simulink model "Marine_LocoMotive_UAV_est_git"  (R2018a)
settings: Solver=ode4  StartTime=0.0  StopTime=40  FixedStep=T  MaxStep=2*T  MinStep=T  RelTol=1e-4
values from neighbouring files (symbols this model uses):
  a_11 = 0.05*m_b    (= 0.625)    [Marine_LocoMotive_UAV_est_git_parameters.m]    (also in Marine_LocoMotive_UAV_medium_est_git_parameters.m = 1.6875; heave_dynamics_chart.m)
  a_33 = m_b    (= 12.5)    [Marine_LocoMotive_UAV_est_git_parameters.m]    (also in Marine_LocoMotive_UAV_medium_est_git_parameters.m = 33.75; heave_dynamics_chart.m)
  A_w = 1*3.3/2    (= 1.65)    [Marine_LocoMotive_UAV_est_git_parameters.m]    (also in Marine_LocoMotive_UAV_medium_est_git_parameters.m = 0.6)
  A_w2 = 1*1.2/2    (= 0.6)    [Marine_LocoMotive_UAV_est_git_parameters.m]    (also in Marine_LocoMotive_UAV_medium_est_git_parameters.m = 0.305)
  Ac = 0.0331    [Marine_LocoMotive_UAV_est_git_parameters.m]    (also in Marine_LocoMotive_UAV_medium_est_git_parameters.m = 0.422)
  alpha_bar = pi/4    (= 0.785398163397)    [Marine_LocoMotive_UAV_est_git_parameters.m]    (also in Marine_LocoMotive_UAV_medium_est_git_parameters.m; heave_dynamics_chart.m = pi/4*sign(V_bar(j)))
  Am = sysd.denominator{1}    [Marine_LocoMotive_UAV_est_git_parameters.m]    (also in Marine_LocoMotive_UAV_medium_est_git_parameters.m)
  Am1_LPF = sysd.denominator{1}    [Marine_LocoMotive_UAV_est_git_parameters.m]    (also in Marine_LocoMotive_UAV_medium_est_git_parameters.m)
  Am2_LPF = sysd.denominator{1}    [Marine_LocoMotive_UAV_est_git_parameters.m]    (also in Marine_LocoMotive_UAV_medium_est_git_parameters.m)
  Am_asw_LPF = sysd.denominator{1}    [Marine_LocoMotive_UAV_est_git_parameters.m]    (also in Marine_LocoMotive_UAV_medium_est_git_parameters.m)
  Am_coup_LPF = sysd.denominator{1}    [Marine_LocoMotive_UAV_est_git_parameters.m]    (also in Marine_LocoMotive_UAV_medium_est_git_parameters.m)
  Am_fast_coup_LPF = sysd.denominator{1}    [Marine_LocoMotive_UAV_est_git_parameters.m]    (also in Marine_LocoMotive_UAV_medium_est_git_parameters.m)
  Am_rdeL_LPF = sysd.denominator{1}    [Marine_LocoMotive_UAV_est_git_parameters.m]    (also in Marine_LocoMotive_UAV_medium_est_git_parameters.m)
  Am_reL_LPF = sysd.denominator{1}    [Marine_LocoMotive_UAV_est_git_parameters.m]    (also in Marine_LocoMotive_UAV_medium_est_git_parameters.m)
  Am_rref20_LPF = sysd.denominator{1}    [Marine_LocoMotive_UAV_est_git_parameters.m]    (also in Marine_LocoMotive_UAV_medium_est_git_parameters.m)
  Am_rref_LPF = sysd.denominator{1}    [Marine_LocoMotive_UAV_est_git_parameters.m]    (also in Marine_LocoMotive_UAV_medium_est_git_parameters.m)
  AmAlpha_LPF = sysd.denominator{1}    [Marine_LocoMotive_UAV_est_git_parameters.m]    (also in Marine_LocoMotive_UAV_medium_est_git_parameters.m)
  Amp_sf = 3    [Marine_LocoMotive_UAV_est_git_parameters.m]    (also in Marine_LocoMotive_UAV_medium_est_git_parameters.m)
  Amp_sf_rp = 0.05*m_u*g    (= 0.8829)    [Marine_LocoMotive_UAV_est_git_parameters.m]    (also in Marine_LocoMotive_UAV_medium_est_git_parameters.m = 9.56475)
  AmV_LPF = sysd.denominator{1}    [Marine_LocoMotive_UAV_est_git_parameters.m]    (also in Marine_LocoMotive_UAV_medium_est_git_parameters.m)
  AmZ_LPF = sysd.denominator{1}    [Marine_LocoMotive_UAV_est_git_parameters.m]    (also in Marine_LocoMotive_UAV_medium_est_git_parameters.m)
  b_11 = 0    [Marine_LocoMotive_UAV_est_git_parameters.m]    (also in Marine_LocoMotive_UAV_medium_est_git_parameters.m; heave_dynamics_chart.m)
  b_33 = 2*m_b*omega_h    (= 19.6349540849)    [Marine_LocoMotive_UAV_est_git_parameters.m]    (also in Marine_LocoMotive_UAV_medium_est_git_parameters.m = 84.8230016469; buoyancy_calc.m = 4.18879020479; heave_dynamics_chart.m = 2*m_b*omega_h)
  Bm = sysd.numerator{1}    [Marine_LocoMotive_UAV_est_git_parameters.m]    (also in Marine_LocoMotive_UAV_medium_est_git_parameters.m)
  Bm1_LPF = sysd.numerator{1}    [Marine_LocoMotive_UAV_est_git_parameters.m]    (also in Marine_LocoMotive_UAV_medium_est_git_parameters.m)
  Bm2_LPF = sysd.numerator{1}    [Marine_LocoMotive_UAV_est_git_parameters.m]    (also in Marine_LocoMotive_UAV_medium_est_git_parameters.m)
  Bm_asw_LPF = sysd.numerator{1}    [Marine_LocoMotive_UAV_est_git_parameters.m]    (also in Marine_LocoMotive_UAV_medium_est_git_parameters.m)
  Bm_coup_LPF = sysd.numerator{1}    [Marine_LocoMotive_UAV_est_git_parameters.m]    (also in Marine_LocoMotive_UAV_medium_est_git_parameters.m)
  Bm_fast_coup_LPF = sysd.numerator{1}    [Marine_LocoMotive_UAV_est_git_parameters.m]    (also in Marine_LocoMotive_UAV_medium_est_git_parameters.m)
  Bm_rdeL_LPF = sysd.numerator{1}    [Marine_LocoMotive_UAV_est_git_parameters.m]    (also in Marine_LocoMotive_UAV_medium_est_git_parameters.m)
  Bm_reL_LPF = sysd.numerator{1}    [Marine_LocoMotive_UAV_est_git_parameters.m]    (also in Marine_LocoMotive_UAV_medium_est_git_parameters.m)
  Bm_rref20_LPF = sysd.numerator{1}    [Marine_LocoMotive_UAV_est_git_parameters.m]    (also in Marine_LocoMotive_UAV_medium_est_git_parameters.m)
  Bm_rref_LPF = sysd.numerator{1}    [Marine_LocoMotive_UAV_est_git_parameters.m]    (also in Marine_LocoMotive_UAV_medium_est_git_parameters.m)
  BmAlpha_LPF = sysd.numerator{1}    [Marine_LocoMotive_UAV_est_git_parameters.m]    (also in Marine_LocoMotive_UAV_medium_est_git_parameters.m)
  BmV_LPF = sysd.numerator{1}    [Marine_LocoMotive_UAV_est_git_parameters.m]    (also in Marine_LocoMotive_UAV_medium_est_git_parameters.m)
  BmZ_LPF = sysd.numerator{1}    [Marine_LocoMotive_UAV_est_git_parameters.m]    (also in Marine_LocoMotive_UAV_medium_est_git_parameters.m)
  C_S = [5;9]*10^-3    [Marine_LocoMotive_UAV_est_git_parameters.m]    (also in Marine_LocoMotive_UAV_medium_est_git_parameters.m; heave_dynamics_chart.m = 0.075/(log10(Re)-2)^2)
  Cd_u = 0.2    [Marine_LocoMotive_UAV_est_git_parameters.m]    (also in Marine_LocoMotive_UAV_medium_est_git_parameters.m)
  D_x = b_11 + D_s(1)    [Marine_LocoMotive_UAV_est_git_parameters.m]    (also in Marine_LocoMotive_UAV_medium_est_git_parameters.m; heave_dynamics_chart.m = b_11 + D_s(i,j))
  D_z = b_33 + D_s(2)    [Marine_LocoMotive_UAV_est_git_parameters.m]    (also in Marine_LocoMotive_UAV_medium_est_git_parameters.m; heave_dynamics_chart.m)
  dc_M_p = 6.7    [Marine_LocoMotive_UAV_est_git_parameters.m]    (also in Marine_LocoMotive_UAV_medium_est_git_parameters.m)
  Delta_h = (A_im/A_b-0.5)*h_b    (= -0.0625)    [Marine_LocoMotive_UAV_est_git_parameters.m]    (also in Marine_LocoMotive_UAV_medium_est_git_parameters.m = -0.075; heave_dynamics_chart.m)
  eps_V = 0.1    [Marine_LocoMotive_UAV_est_git_parameters.m]    (also in Marine_LocoMotive_UAV_medium_est_git_parameters.m)
  epsilon_1 = 5    [Marine_LocoMotive_UAV_est_git_parameters.m]    (also in Marine_LocoMotive_UAV_medium_est_git_parameters.m)
  epsilon_e_u1 = 0.05    [Marine_LocoMotive_UAV_est_git_parameters.m]    (also in Marine_LocoMotive_UAV_medium_est_git_parameters.m)
  epsilon_w = 0    [Marine_LocoMotive_UAV_est_git_parameters.m]    (also in Marine_LocoMotive_UAV_medium_est_git_parameters.m)
  epsilon_w2 = pi    (= 3.14159265359)    [Marine_LocoMotive_UAV_est_git_parameters.m]    (also in Marine_LocoMotive_UAV_medium_est_git_parameters.m)
  g = 9.81    [Marine_LocoMotive_UAV_est_git_parameters.m]    (also in Marine_LocoMotive_UAV_medium_est_git_parameters.m; heave_dynamics_chart.m)
  gamma_d_p = (2*0.3/0.03*2*0.2*12/4)/10    (= 2.4)    [Marine_LocoMotive_UAV_est_git_parameters.m]    (also in Marine_LocoMotive_UAV_medium_est_git_parameters.m)
  H = 10    [Marine_LocoMotive_UAV_est_git_parameters.m]    (also in Marine_LocoMotive_UAV_medium_est_git_parameters.m)
  h_b = 0.25    [Marine_LocoMotive_UAV_est_git_parameters.m]    (also in Marine_LocoMotive_UAV_medium_est_git_parameters.m = 0.3; buoyancy_calc.m = 0.15; heave_dynamics_chart.m)
  J_b = m_b*h_b*l_b/12    (= 0.208333333333)    [Marine_LocoMotive_UAV_est_git_parameters.m]    (also in Marine_LocoMotive_UAV_medium_est_git_parameters.m = 1.265625; heave_dynamics_chart.m)
  J_u = 0.03    [Marine_LocoMotive_UAV_est_git_parameters.m]    (also in Marine_LocoMotive_UAV_medium_est_git_parameters.m = 1.51708333333)
  K = 40    [Marine_LocoMotive_UAV_est_git_parameters.m]    (also in Marine_LocoMotive_UAV_medium_est_git_parameters.m = 83.3333333333)
  k3 = 24    [Marine_LocoMotive_UAV_est_git_parameters.m]    (also in Marine_LocoMotive_UAV_medium_est_git_parameters.m)
  k4 = 0.8    [Marine_LocoMotive_UAV_est_git_parameters.m]    (also in Marine_LocoMotive_UAV_medium_est_git_parameters.m)
  k_w = omega_w^2/g    (= 0.0628797426165)    [Marine_LocoMotive_UAV_est_git_parameters.m]    (also in Marine_LocoMotive_UAV_medium_est_git_parameters.m = 0.160972141098; heave_dynamics_chart.m = omega_w^2/g)
  k_w2 = omega_w2^2/g    (= 0.160972141098)    [Marine_LocoMotive_UAV_est_git_parameters.m]    (also in Marine_LocoMotive_UAV_medium_est_git_parameters.m = 0.251518970466)
  kd_a = 5.6    [Marine_LocoMotive_UAV_est_git_parameters.m]    (also in Marine_LocoMotive_UAV_medium_est_git_parameters.m)
  kd_r = 19.5    [Marine_LocoMotive_UAV_est_git_parameters.m]    (also in Marine_LocoMotive_UAV_medium_est_git_parameters.m)
  kd_t = 10    [Marine_LocoMotive_UAV_est_git_parameters.m]    (also in Marine_LocoMotive_UAV_medium_est_git_parameters.m = 25)
  kd_x = 5    [Marine_LocoMotive_UAV_est_git_parameters.m]    (also in Marine_LocoMotive_UAV_medium_est_git_parameters.m)
  kd_z = 2    [Marine_LocoMotive_UAV_est_git_parameters.m]    (also in Marine_LocoMotive_UAV_medium_est_git_parameters.m)
  ki_a = 1.6    [Marine_LocoMotive_UAV_est_git_parameters.m]    (also in Marine_LocoMotive_UAV_medium_est_git_parameters.m)
  ki_r = 9    [Marine_LocoMotive_UAV_est_git_parameters.m]    (also in Marine_LocoMotive_UAV_medium_est_git_parameters.m)
  ki_T = 12    [Marine_LocoMotive_UAV_est_git_parameters.m]    (also in Marine_LocoMotive_UAV_medium_est_git_parameters.m)
  ki_x = 1.2    [Marine_LocoMotive_UAV_est_git_parameters.m]    (also in Marine_LocoMotive_UAV_medium_est_git_parameters.m)
  ki_z = 1    [Marine_LocoMotive_UAV_est_git_parameters.m]    (also in Marine_LocoMotive_UAV_medium_est_git_parameters.m)
  kp_a = 9.6    [Marine_LocoMotive_UAV_est_git_parameters.m]    (also in Marine_LocoMotive_UAV_medium_est_git_parameters.m)
  kp_r = 45    [Marine_LocoMotive_UAV_est_git_parameters.m]    (also in Marine_LocoMotive_UAV_medium_est_git_parameters.m)
  kp_t = 20    [Marine_LocoMotive_UAV_est_git_parameters.m]    (also in Marine_LocoMotive_UAV_medium_est_git_parameters.m = 50)
  kp_T = 25    [Marine_LocoMotive_UAV_est_git_parameters.m]    (also in Marine_LocoMotive_UAV_medium_est_git_parameters.m)
  kp_x = 7    [Marine_LocoMotive_UAV_est_git_parameters.m]    (also in Marine_LocoMotive_UAV_medium_est_git_parameters.m)
  kp_z = 3    [Marine_LocoMotive_UAV_est_git_parameters.m]    (also in Marine_LocoMotive_UAV_medium_est_git_parameters.m)
  L = 0.2    [Marine_LocoMotive_UAV_est_git_parameters.m]    (also in Marine_LocoMotive_UAV_medium_est_git_parameters.m = 0.8)
  l_b = 0.8    [Marine_LocoMotive_UAV_est_git_parameters.m]    (also in Marine_LocoMotive_UAV_medium_est_git_parameters.m = 1.5; buoyancy_calc.m = 0.5; heave_dynamics_chart.m)
  Lc_0 = 7    [Marine_LocoMotive_UAV_est_git_parameters.m]    (also in Marine_LocoMotive_UAV_medium_est_git_parameters.m = 20)
  LIMIT_CMD_PITCH = 45*pi/180    (= 0.785398163397)    [Marine_LocoMotive_UAV_est_git_parameters.m]    (also in Marine_LocoMotive_UAV_medium_est_git_parameters.m)
  LIMIT_uCMD_HEIGHT = 0.9*n_motors*K    (= 144)    [Marine_LocoMotive_UAV_est_git_parameters.m]    (also in Marine_LocoMotive_UAV_medium_est_git_parameters.m = 450)
  m_b = rho_w*Vol_b/4    (= 12.5)    [Marine_LocoMotive_UAV_est_git_parameters.m]    (also in Marine_LocoMotive_UAV_medium_est_git_parameters.m = 33.75; buoyancy_calc.m = 5; heave_dynamics_chart.m)
  m_u = 1.8    [Marine_LocoMotive_UAV_est_git_parameters.m]    (also in Marine_LocoMotive_UAV_medium_est_git_parameters.m = 19.5)
  min_sf = 5    [Marine_LocoMotive_UAV_est_git_parameters.m]    (also in Marine_LocoMotive_UAV_medium_est_git_parameters.m)
  min_sf_rp = 0.35*m_u*g    (= 6.1803)    [Marine_LocoMotive_UAV_est_git_parameters.m]    (also in Marine_LocoMotive_UAV_medium_est_git_parameters.m = 66.95325)
  n_motors = 4    [Marine_LocoMotive_UAV_est_git_parameters.m]    (also in Marine_LocoMotive_UAV_medium_est_git_parameters.m = 6)
  nu_w = 1.787*10^-6    (= 1.787e-06)    [Marine_LocoMotive_UAV_est_git_parameters.m]    (also in Marine_LocoMotive_UAV_medium_est_git_parameters.m; buoyancy_calc.m; heave_dynamics_chart.m)
  omega_w = 2*pi/T_w    (= 0.785398163397)    [Marine_LocoMotive_UAV_est_git_parameters.m]    (also in Marine_LocoMotive_UAV_medium_est_git_parameters.m = 1.25663706144; heave_dynamics_chart.m = 2*pi/T_i)
  omega_w2 = 2*pi/T_w2    (= 1.25663706144)    [Marine_LocoMotive_UAV_est_git_parameters.m]    (also in Marine_LocoMotive_UAV_medium_est_git_parameters.m = 1.57079632679)
  r_0 = sqrt( (X0_b(1) - X0_u(1))^2 +(X0_b(2) - X0_u(2))^2 )    [Marine_LocoMotive_UAV_est_git_parameters.m]    (also in Marine_LocoMotive_UAV_medium_est_git_parameters.m)
  R_b = 0.1    [buoyancy_calc.m]
  r_bar = Lc_0-0.3    (= 6.7)    [Marine_LocoMotive_UAV_est_git_parameters.m]    (also in Marine_LocoMotive_UAV_medium_est_git_parameters.m = 19.7)
  r_min = (zu_bar-H)-0.2    [Marine_LocoMotive_UAV_est_git_parameters.m]    (also in Marine_LocoMotive_UAV_medium_est_git_parameters.m)
  rho_a = 1.225    [Marine_LocoMotive_UAV_est_git_parameters.m]    (also in Marine_LocoMotive_UAV_medium_est_git_parameters.m)
  rho_w = 1000    [Marine_LocoMotive_UAV_est_git_parameters.m]    (also in Marine_LocoMotive_UAV_medium_est_git_parameters.m; buoyancy_calc.m; heave_dynamics_chart.m)
  T = 1/500    (= 0.002)    [Marine_LocoMotive_UAV_est_git_parameters.m]    (also in Marine_LocoMotive_UAV_medium_est_git_parameters.m)
  T_init = 10    [Marine_LocoMotive_UAV_est_git_parameters.m]    (also in Marine_LocoMotive_UAV_medium_est_git_parameters.m)
  Theta0 = 0    [Marine_LocoMotive_UAV_est_git_parameters.m]    (also in Marine_LocoMotive_UAV_medium_est_git_parameters.m)
  torque_corr = 2*cosd(60)+1    [Marine_LocoMotive_UAV_est_git_parameters.m]    (also in Marine_LocoMotive_UAV_medium_est_git_parameters.m)
  u_s = w_dir*A_w^2*omega_w*k_w*exp(2*k_w*(-Delta_h/2))    [Marine_LocoMotive_UAV_est_git_parameters.m]    (also in Marine_LocoMotive_UAV_medium_est_git_parameters.m)
  u_s2 = w_dir2*A_w2^2*omega_w2*k_w2*exp(2*k_w2*(-Delta_h/2))    [Marine_LocoMotive_UAV_est_git_parameters.m]    (also in Marine_LocoMotive_UAV_medium_est_git_parameters.m)
  u_t = -1*0.5*1    (= -0.5)    [Marine_LocoMotive_UAV_est_git_parameters.m]    (also in Marine_LocoMotive_UAV_medium_est_git_parameters.m)
  u_w = 0*0.2    (= 0)    [Marine_LocoMotive_UAV_est_git_parameters.m]    (also in Marine_LocoMotive_UAV_medium_est_git_parameters.m)
  V0_b = [u_t+u_w+u_s+v_x_w, v_z_w].*[1 1]    [Marine_LocoMotive_UAV_est_git_parameters.m]    (also in Marine_LocoMotive_UAV_medium_est_git_parameters.m = [u_t+u_w+u_s+v_x_w, v_z_w])
  V0_u = V0_b    [Marine_LocoMotive_UAV_est_git_parameters.m]    (also in Marine_LocoMotive_UAV_medium_est_git_parameters.m = [0 0])
  V_bar = 4    [Marine_LocoMotive_UAV_est_git_parameters.m]    (also in Marine_LocoMotive_UAV_medium_est_git_parameters.m; heave_dynamics_chart.m = [-20:0.1:20]')
  Vol_b = A_b*l_b    (= 0.05)    [Marine_LocoMotive_UAV_est_git_parameters.m]    (also in Marine_LocoMotive_UAV_medium_est_git_parameters.m = 0.135; heave_dynamics_chart.m)
  w_dir = 1    [Marine_LocoMotive_UAV_est_git_parameters.m]    (also in Marine_LocoMotive_UAV_medium_est_git_parameters.m; heave_dynamics_chart.m)
  w_dir2 = 1    [Marine_LocoMotive_UAV_est_git_parameters.m]    (also in Marine_LocoMotive_UAV_medium_est_git_parameters.m)
  X0_b = [0,H-Delta_h]    [Marine_LocoMotive_UAV_est_git_parameters.m]    (also in Marine_LocoMotive_UAV_medium_est_git_parameters.m)
  X0_u = X0_b + [3/7 3/7]*Lc_0    [Marine_LocoMotive_UAV_est_git_parameters.m]    (also in Marine_LocoMotive_UAV_medium_est_git_parameters.m)
  zu_bar = X0_b(2) + Lc_0*sin(alpha_bar_0)    [Marine_LocoMotive_UAV_est_git_parameters.m]    (also in Marine_LocoMotive_UAV_medium_est_git_parameters.m)
undefined symbols (not defined in the file or in its folder): Am_HPF, Am_LPF, Am_LPF2, an1, an1_v, an2, an3, Bm_HPF, Bm_LPF, Bm_LPF2, bn1, bn1_v, bn2, bn3, DiscIntNeverNeededParam, F, Light, magnitude, MIL, OMEGA_FILTER_OUTER, Tc, Tg, Tn, Ts, Tsc, Tz, X_GPS_offset
libraries: simulink x55, simulink_extras x9, aerolibwind2 x2
(part 8 of 9)

== system Marine_LocoMotive_UAV_est_git/UAV controller/u_a_Lyapunov/Subsystem1/alpha 0 ==
  X : Inport
  Trigger : TriggerPort  VariantControl=Variant
  Xu_init : Outport
  wires:
  X/1 -> Xu_init/1

== system Marine_LocoMotive_UAV_est_git/UAV controller/u_a_Lyapunov/Subsystem1/cond1 ==
  r : Inport
  r_dot : Inport  Port=2
  coupled : Inport  Port=3
  Constant : Constant  Value=Lc_0
  Constant2 : Constant  Value=T
  MATLAB Function : MATLAB Function  TreatAsAtomicUnit=on
  r_dot filt2 : Scope
  key : Outport
  wires:
  r/1 -> MATLAB Function/1(r)
  Constant/1 -> MATLAB Function/4(Lc)
  Constant2/1 -> MATLAB Function/5(dt)
  MATLAB Function/1(y) -> key/1
  r_dot/1 -> MATLAB Function/2(r_dot)
  coupled/1 -> MATLAB Function/3(coupled)
  MATLAB Function/2(t) -> r_dot filt2/1

== system Marine_LocoMotive_UAV_est_git/UAV controller/u_r_V_Lyapunov buoy velocity/Smooth channel switching1/C1 transition ==
  C1 : Inport
  switch : Inport  Port=2
  C2_0 : Inport  Port=3
  Compare To Constant : simulink/Logic and Bit Operations/Compare To Constant  relop=<  const=0.01  OutDataTypeStr=boolean
  Constant : Constant
  Constant1 : Constant  Value=0.01
  Delay1 : Delay  DelayLength=1
  IC : InitialCondition  Value=0
  Logical Operator : Logic  Operator=NOT  AllPortsSameDT=off  OutDataTypeStr=boolean
  Product : Product
  Subsystem : Subsystem
  Sum : Sum  Inputs=-+|
  Sum1 : Sum  Inputs=++|
  Sum3 : Sum  Inputs=|++
  Switch1 : Switch  Criteria=u2 > Threshold  Threshold=0.5
  Switch2 : Switch  Criteria=u2 > Threshold  Threshold=0.5
  latch : Subsystem  TreatAsAtomicUnit=on
  latch error ON : Scope
  record C2_0 : Subsystem  TreatAsAtomicUnit=on
  smooth transition to C1 : Subsystem  TreatAsAtomicUnit=on
  trigger and reset latch : Subsystem
  C1_trans : Outport
  wires:
  trigger and reset latch/1(Out1) -> latch/Trigger
  Logical Operator/1 -> Product/2
  IC/1 -> latch/1(In1), trigger and reset latch/2(In2)
  switch/1 -> smooth transition to C1/Enable, Subsystem/Enable, trigger and reset latch/1(In1), record C2_0/Trigger, Delay1/1, Logical Operator/1, Switch2/2
  Sum/1 -> smooth transition to C1/1(In1)
  Delay1/1 -> smooth transition to C1/2(reset)
  Compare To Constant/1 -> IC/1
  Subsystem/1(Out1) -> Sum3/1
  Sum3/1 -> Compare To Constant/1
  Product/1 -> Sum3/2  "do not latch C1 is off"
  Constant1/1 -> Product/1
  Constant/1 -> Switch2/3
  Switch2/1 -> latch error ON/1, Switch1/2
  latch/1(Out1) -> Switch2/1
  Switch1/1 -> C1_trans/1  "out"
  C1/1 -> Sum/2, Switch1/1, Subsystem/2(C1)  "C1"
  record C2_0/1(Out1) -> Sum1/1, Sum/1  "C2_0"
  smooth transition to C1/1(Out1) -> Sum1/2
  C2_0/1 -> record C2_0/1(In1)
  Sum1/1 -> Switch1/3, Subsystem/1(addition with C2_0)  "addition with C2_0"

== system Marine_LocoMotive_UAV_est_git/UAV controller/u_r_V_Lyapunov buoy velocity/Smooth channel switching1/C2 transition ==
  C2 : Inport
  switch : Inport  Port=2
  C1_0 : Inport  Port=3
  Compare To Constant : simulink/Logic and Bit Operations/Compare To Constant  relop=<  const=0.01  OutDataTypeStr=boolean
  Constant : Constant
  Constant1 : Constant  Value=0.01
  Delay1 : Delay  DelayLength=1
  Logical Operator : Logic  Operator=NOT  AllPortsSameDT=off  OutDataTypeStr=boolean
  Product : Product
  Subsystem : Subsystem
  Sum : Sum  Inputs=-+|
  Sum1 : Sum  Inputs=++|
  Sum3 : Sum  Inputs=|++
  Switch1 : Switch  Criteria=u2 > Threshold  Threshold=0.5
  Switch2 : Switch  Criteria=u2 > Threshold  Threshold=0.5
  latch : Subsystem  TreatAsAtomicUnit=on
  latch error ON : Scope
  record C1_0 : Subsystem  TreatAsAtomicUnit=on
  smooth transition to C1 : Subsystem  TreatAsAtomicUnit=on
  trigger and reset latch : Subsystem
  C2_trans : Outport
  wires:
  trigger and reset latch/1(Out1) -> latch/Trigger
  Compare To Constant/1 -> latch/1(In1), trigger and reset latch/2(In2)
  Subsystem/1(Out1) -> Sum3/1
  Delay1/1 -> smooth transition to C1/2(reset)
  Logical Operator/1 -> Product/2
  Sum3/1 -> Compare To Constant/1
  Constant1/1 -> Product/1
  Product/1 -> Sum3/2
  latch/1(Out1) -> Switch2/1
  Constant/1 -> Switch2/3
  Sum1/1 -> Switch1/3, Subsystem/1(addition with C1_0)  "addition with C1_0"
  C1_0/1 -> record C1_0/1(In1)
  smooth transition to C1/1(Out1) -> Sum1/2
  record C1_0/1(Out1) -> Sum/1, Sum1/1  "C1_0"
  switch/1 -> record C1_0/Trigger, trigger and reset latch/1(trigger), Subsystem/Enable, smooth transition to C1/Enable, Delay1/1, Logical Operator/1, Switch2/2  "trigger"
  Switch2/1 -> latch error ON/1, Switch1/2
  C2/1 -> Switch1/1, Subsystem/2(C2), Sum/2  "C2"
  Switch1/1 -> C2_trans/1  "out"
  Sum/1 -> smooth transition to C1/1(In1)

== system Marine_LocoMotive_UAV_est_git/Quadrotor+buoy/3-DOF equations of motion Earth frame/D_123/Water Daming/rotation matrix R body to earth ==
  angle (rad) : Inport
  Gain : Gain  Gain=-1
  Signal Specification1 : SignalSpecification  Dimensions=2
  Signal Specification2 : SignalSpecification  Dimensions=2
  Trigonometric Function1 : Trigonometry  Operator=sincos
  Vector Concatenate1 : Concatenate  Mode=Multidimensional array  ConcatenateDimension=2
  Vector Concatenate2 : Concatenate
  Vector Concatenate3 : Concatenate
  R : Outport
  wires:
  Gain/1 -> Vector Concatenate3/1
  Trigonometric Function1/1 -> Gain/1, Vector Concatenate2/2
  Trigonometric Function1/2 -> Vector Concatenate2/1, Vector Concatenate3/2
  angle (rad)/1 -> Trigonometric Function1/1
  Vector Concatenate3/1 -> Signal Specification2/1
  Vector Concatenate2/1 -> Signal Specification1/1
  Vector Concatenate1/1 -> R/1
  Signal Specification1/1 -> Vector Concatenate1/1
  Signal Specification2/1 -> Vector Concatenate1/2

== system Marine_LocoMotive_UAV_est_git/Quadrotor+buoy/3-DOF equations of motion Earth frame/Quadrotor Dynamics Outer-Loop/quadrotor position from relative buoy-UAV position/rotation matrix R  ==
  angle (rad) : Inport
  Gain2 : Gain  Gain=-1
  Gain3 : Gain  Gain=-1
  Signal Specification1 : SignalSpecification  Dimensions=2
  Signal Specification2 : SignalSpecification  Dimensions=2
  Trigonometric Function1 : Trigonometry  Operator=sincos
  Vector Concatenate1 : Concatenate  Mode=Multidimensional array  ConcatenateDimension=2
  Vector Concatenate2 : Concatenate
  Vector Concatenate3 : Concatenate
  R : Outport
  wires:
  Signal Specification2/1 -> Vector Concatenate1/2
  Signal Specification1/1 -> Vector Concatenate1/1
  Vector Concatenate1/1 -> R/1
  Vector Concatenate2/1 -> Signal Specification1/1
  Vector Concatenate3/1 -> Signal Specification2/1
  angle (rad)/1 -> Trigonometric Function1/1
  Trigonometric Function1/1 -> Gain3/1
  Trigonometric Function1/2 -> Vector Concatenate3/2, Gain2/1
  Gain3/1 -> Vector Concatenate2/2, Vector Concatenate3/1
  Gain2/1 -> Vector Concatenate2/1

== system Marine_LocoMotive_UAV_est_git/Quadrotor+buoy/3-DOF equations of motion Earth frame/azimuthal dynamics/Coupled System's azimuthal dynamics/azimuth angle dynamics in the coupled system ==
  alpha_ddot : Inport
  alpha init : Inport  Port=2
  alpha dot init : Inport  Port=3
  reset : Inport  Port=4
  Enable : EnablePort
  " alpha" : Scope
  " alpha dot" : Scope
  " alpha dot init" : Scope
  " alpha init" : Scope
  alpha : DiscreteIntegrator  IntegratorMethod=Integration: Backward Euler  ExternalReset=level  InitialConditionSource=external  InitialCondition=alpha_0  SampleTime=-1  ICPrevOutput=DiscIntNeverNeededParam  ICPrevScaledInput=DiscIntNeverNeededParam
  dot(alpha) : DiscreteIntegrator  IntegratorMethod=Integration: Backward Euler  ExternalReset=level  InitialConditionSource=external  SampleTime=-1  ICPrevOutput=DiscIntNeverNeededParam  ICPrevScaledInput=DiscIntNeverNeededParam
  "reset " : Scope
  "alpha " : Outport
  alpha dot : Outport  Port=2
  wires:
  dot(alpha)/1 -> alpha/1, " alpha dot"/1, alpha dot/1
  alpha_ddot/1 -> dot(alpha)/1
  alpha/1 -> "alpha "/1, " alpha"/1
  alpha dot init/1 -> " alpha dot init"/1, dot(alpha)/3
  alpha init/1 -> " alpha init"/1, alpha/3
  reset/1 -> "reset "/1, alpha/2, dot(alpha)/2

== system Marine_LocoMotive_UAV_est_git/Quadrotor+buoy/3-DOF equations of motion Earth frame/azimuthal dynamics/Coupled System's azimuthal dynamics/get initial azimuth angle for the coupled dynamics ==
  alpha decoupled : Inport
  alpha dot decoupled : Inport  Port=2
  Trigger : TriggerPort  VariantControl=Variant
  alpha init : Outport
  alpha dot init : Outport  Port=2
  wires:
  alpha decoupled/1 -> alpha init/1
  alpha dot decoupled/1 -> alpha dot init/1

== system Marine_LocoMotive_UAV_est_git/Quadrotor+buoy/3-DOF equations of motion Earth frame/azimuthal dynamics/Decoupled System's azimuthal dynamics/magnitude ==
  dX : Inport
  Math Function2 : Math  Operator=square  SaturateOnIntegerOverflow=on
  Sqrt : Sqrt  SaturateOnIntegerOverflow=on
  Sum of Elements : Sum  Inputs=+
  r : Outport
  wires:
  Math Function2/1 -> Sum of Elements/1
  Sum of Elements/1 -> Sqrt/1
  dX/1 -> Math Function2/1
  Sqrt/1 -> r/1

== system Marine_LocoMotive_UAV_est_git/Quadrotor+buoy/3-DOF equations of motion Earth frame/azimuthal dynamics/Decoupled System's azimuthal dynamics/rotation matrix R  ==
  angle (rad) : Inport
  Gain : Gain  Gain=-1
  Signal Specification1 : SignalSpecification  Dimensions=2
  Signal Specification2 : SignalSpecification  Dimensions=2
  Trigonometric Function1 : Trigonometry  Operator=sincos
  Vector Concatenate1 : Concatenate  Mode=Multidimensional array  ConcatenateDimension=2
  Vector Concatenate2 : Concatenate
  Vector Concatenate3 : Concatenate
  R : Outport
  wires:
  Signal Specification2/1 -> Vector Concatenate1/2
  Signal Specification1/1 -> Vector Concatenate1/1
  Vector Concatenate1/1 -> R/1
  Vector Concatenate2/1 -> Signal Specification1/1
  Vector Concatenate3/1 -> Signal Specification2/1
  angle (rad)/1 -> Trigonometric Function1/1
  Trigonometric Function1/2 -> Vector Concatenate3/2, Vector Concatenate2/1
  Trigonometric Function1/1 -> Vector Concatenate2/2, Gain/1
  Gain/1 -> Vector Concatenate3/1

== system Marine_LocoMotive_UAV_est_git/Quadrotor+buoy/3-DOF equations of motion Earth frame/azimuthal dynamics/Decoupled System's azimuthal dynamics/rotation matrix R 1 ==
  angle (rad) : Inport
  Gain : Gain  Gain=-1
  Signal Specification1 : SignalSpecification  Dimensions=2
  Signal Specification2 : SignalSpecification  Dimensions=2
  Trigonometric Function1 : Trigonometry  Operator=sincos
  Vector Concatenate1 : Concatenate  Mode=Multidimensional array  ConcatenateDimension=2
  Vector Concatenate2 : Concatenate
  Vector Concatenate3 : Concatenate
  R : Outport
  wires:
  Gain/1 -> Vector Concatenate3/1
  Trigonometric Function1/1 -> Gain/1, Vector Concatenate2/2
  Trigonometric Function1/2 -> Vector Concatenate2/1, Vector Concatenate3/2
  angle (rad)/1 -> Trigonometric Function1/1
  Vector Concatenate3/1 -> Signal Specification2/1
  Vector Concatenate2/1 -> Signal Specification1/1
  Vector Concatenate1/1 -> R/1
  Signal Specification1/1 -> Vector Concatenate1/1
  Signal Specification2/1 -> Vector Concatenate1/2

== system Marine_LocoMotive_UAV_est_git/Sensors and Filters/Sensors/ Sonar (10Hz) (true elevation instead real sonar signal)/Sampler/Triggered Subsystem ==
  In1 : Inport
  Trigger : TriggerPort  VariantControl=(inherit)
  Out1 : Outport
  wires:
  In1/1 -> Out1/1

== system Marine_LocoMotive_UAV_est_git/UAV controller/switch controllers/Smooth channel switching/C1 transition/Subsystem ==
  addition with C2_0 : Inport
  C1 : Inport  Port=2
  Enable : EnablePort
  Abs : Abs
  Sum2 : Sum  Inputs=-+|
  Out1 : Outport
  wires:
  addition with C2_0/1 -> Sum2/1
  C1/1 -> Sum2/2
  Sum2/1 -> Abs/1  "calculate the error"
  Abs/1 -> Out1/1

== system Marine_LocoMotive_UAV_est_git/UAV controller/switch controllers/Smooth channel switching/C1 transition/latch ==
  In1 : Inport
  Trigger : TriggerPort  VariantControl=Variant
  Out1 : Outport
  wires:
  In1/1 -> Out1/1

== system Marine_LocoMotive_UAV_est_git/UAV controller/switch controllers/Smooth channel switching/C1 transition/record C2_0 ==
  In1 : Inport
  Trigger : TriggerPort  TriggerType=either  VariantControl=Variant
  Out1 : Outport
  wires:
  In1/1 -> Out1/1

== system Marine_LocoMotive_UAV_est_git/UAV controller/switch controllers/Smooth channel switching/C1 transition/smooth transition to C1 ==
  In1 : Inport
  reset : Inport  Port=2
  Enable : EnablePort
  Discrete Transfer Fcn1 : DiscreteTransferFcn  Numerator=Bm_coup_LPF  Denominator=Am_coup_LPF  ExternalReset=Either
      settings: InputPortMap=u0,r7
  Out1 : Outport
  wires:
  Discrete Transfer Fcn1/1 -> Out1/1
  In1/1 -> Discrete Transfer Fcn1/1
  reset/1 -> Discrete Transfer Fcn1/2

== system Marine_LocoMotive_UAV_est_git/UAV controller/switch controllers/Smooth channel switching/C1 transition/trigger and reset latch ==
  In1 : Inport
  In2 : Inport  Port=2
  Abs : Abs
  Add : Sum
  Data Type Conversion : DataTypeConversion
  Data Type Conversion1 : DataTypeConversion
  Discrete Derivative1 : simulink/Discrete/Discrete Derivative  gainval=1.0  ICPrevScaledInput=0.0  OutMin=[]  OutMax=[]  OutDataType=fixdt(1, 16)  OutScaling=2^-10  DoSatur=off
  IC1 : InitialCondition  Value=0
  Saturation : Saturate  UpperLimit=1  LowerLimit=0
  Out1 : Outport
  wires:
  IC1/1 -> Saturation/1
  Discrete Derivative1/1 -> Abs/1
  In2/1 -> Data Type Conversion/1
  Abs/1 -> IC1/1
  Add/1 -> Out1/1
  Data Type Conversion1/1 -> Discrete Derivative1/1
  Saturation/1 -> Add/1
  Data Type Conversion/1 -> Add/2
  In1/1 -> Data Type Conversion1/1

== system Marine_LocoMotive_UAV_est_git/UAV controller/switch controllers/Smooth channel switching/C2 transition/Subsystem ==
  addition with C1_0 : Inport
  C2 : Inport  Port=2
  Enable : EnablePort
  Abs : Abs
  Sum2 : Sum  Inputs=-+|
  Out1 : Outport
  wires:
  addition with C1_0/1 -> Sum2/1
  Sum2/1 -> Abs/1  "calculate the error"
  Abs/1 -> Out1/1
  C2/1 -> Sum2/2

== system Marine_LocoMotive_UAV_est_git/UAV controller/switch controllers/Smooth channel switching/C2 transition/latch ==
  In1 : Inport
  Trigger : TriggerPort  VariantControl=Variant
  Out1 : Outport
  wires:
  In1/1 -> Out1/1

== system Marine_LocoMotive_UAV_est_git/UAV controller/switch controllers/Smooth channel switching/C2 transition/record C1_0 ==
  In1 : Inport
  Trigger : TriggerPort  VariantControl=Variant
  Out1 : Outport
  wires:
  In1/1 -> Out1/1

== system Marine_LocoMotive_UAV_est_git/UAV controller/switch controllers/Smooth channel switching/C2 transition/smooth transition to C1 ==
  In1 : Inport
  reset : Inport  Port=2
  Enable : EnablePort
  Discrete Transfer Fcn1 : DiscreteTransferFcn  Numerator=Bm_coup_LPF  Denominator=Am_coup_LPF  ExternalReset=Either
      settings: InputPortMap=u0,r7
  Out1 : Outport
  wires:
  Discrete Transfer Fcn1/1 -> Out1/1
  In1/1 -> Discrete Transfer Fcn1/1
  reset/1 -> Discrete Transfer Fcn1/2

== system Marine_LocoMotive_UAV_est_git/UAV controller/switch controllers/Smooth channel switching/C2 transition/trigger and reset latch ==
  trigger : Inport
  In2 : Inport  Port=2
  Abs : Abs
  Add : Sum
  Data Type Conversion : DataTypeConversion
  Data Type Conversion1 : DataTypeConversion
  Discrete Derivative1 : simulink/Discrete/Discrete Derivative  gainval=1.0  ICPrevScaledInput=0.0  OutMin=[]  OutMax=[]  OutDataType=fixdt(1, 16)  OutScaling=2^-10  DoSatur=off
  IC1 : InitialCondition  Value=0
  Saturation : Saturate  UpperLimit=1  LowerLimit=0
  Out1 : Outport
  wires:
  trigger/1 -> Data Type Conversion1/1
  Add/1 -> Out1/1
  Abs/1 -> IC1/1
  Data Type Conversion/1 -> Add/2
  In2/1 -> Data Type Conversion/1
  Saturation/1 -> Add/1
  Discrete Derivative1/1 -> Abs/1
  Data Type Conversion1/1 -> Discrete Derivative1/1
  IC1/1 -> Saturation/1

== system Marine_LocoMotive_UAV_est_git/UAV controller/u_r_V_Lyapunov buoy velocity/Smooth channel switching1/C1 transition/Subsystem ==
  addition with C2_0 : Inport
  C1 : Inport  Port=2
  Enable : EnablePort
  Abs : Abs
  Sum2 : Sum  Inputs=-+|
  Out1 : Outport
  wires:
  Abs/1 -> Out1/1
  Sum2/1 -> Abs/1  "calculate the error"
  C1/1 -> Sum2/2
  addition with C2_0/1 -> Sum2/1

== system Marine_LocoMotive_UAV_est_git/UAV controller/u_r_V_Lyapunov buoy velocity/Smooth channel switching1/C1 transition/latch ==
  In1 : Inport
  Trigger : TriggerPort  VariantControl=Variant
  Out1 : Outport
  wires:
  In1/1 -> Out1/1

== system Marine_LocoMotive_UAV_est_git/UAV controller/u_r_V_Lyapunov buoy velocity/Smooth channel switching1/C1 transition/record C2_0 ==
  In1 : Inport
  Trigger : TriggerPort  TriggerType=either  VariantControl=Variant
  Out1 : Outport
  wires:
  In1/1 -> Out1/1

== system Marine_LocoMotive_UAV_est_git/UAV controller/u_r_V_Lyapunov buoy velocity/Smooth channel switching1/C1 transition/smooth transition to C1 ==
  In1 : Inport
  reset : Inport  Port=2
  Enable : EnablePort
  Discrete Transfer Fcn1 : DiscreteTransferFcn  Numerator=Bm_coup_LPF  Denominator=Am_coup_LPF  ExternalReset=Either
      settings: InputPortMap=u0,r7
  Out1 : Outport
  wires:
  reset/1 -> Discrete Transfer Fcn1/2
  In1/1 -> Discrete Transfer Fcn1/1
  Discrete Transfer Fcn1/1 -> Out1/1

== system Marine_LocoMotive_UAV_est_git/UAV controller/u_r_V_Lyapunov buoy velocity/Smooth channel switching1/C1 transition/trigger and reset latch ==
  In1 : Inport
  In2 : Inport  Port=2
  Abs : Abs
  Add : Sum
  Data Type Conversion : DataTypeConversion
  Data Type Conversion1 : DataTypeConversion
  Discrete Derivative1 : simulink/Discrete/Discrete Derivative  gainval=1.0  ICPrevScaledInput=0.0  OutMin=[]  OutMax=[]  OutDataType=fixdt(1, 16)  OutScaling=2^-10  DoSatur=off
  IC1 : InitialCondition  Value=0
  Saturation : Saturate  UpperLimit=1  LowerLimit=0
  Out1 : Outport
  wires:
  In1/1 -> Data Type Conversion1/1
  Data Type Conversion/1 -> Add/2
  Saturation/1 -> Add/1
  Data Type Conversion1/1 -> Discrete Derivative1/1
  Add/1 -> Out1/1
  Abs/1 -> IC1/1
  In2/1 -> Data Type Conversion/1
  Discrete Derivative1/1 -> Abs/1
  IC1/1 -> Saturation/1

== system Marine_LocoMotive_UAV_est_git/UAV controller/u_r_V_Lyapunov buoy velocity/Smooth channel switching1/C2 transition/Subsystem ==
  addition with C1_0 : Inport
  C2 : Inport  Port=2
  Enable : EnablePort
  Abs : Abs
  Sum2 : Sum  Inputs=-+|
  Out1 : Outport
  wires:
  C2/1 -> Sum2/2
  Abs/1 -> Out1/1
  Sum2/1 -> Abs/1  "calculate the error"
  addition with C1_0/1 -> Sum2/1

== system Marine_LocoMotive_UAV_est_git/UAV controller/u_r_V_Lyapunov buoy velocity/Smooth channel switching1/C2 transition/latch ==
  In1 : Inport
  Trigger : TriggerPort  VariantControl=Variant
  Out1 : Outport
  wires:
  In1/1 -> Out1/1

== system Marine_LocoMotive_UAV_est_git/UAV controller/u_r_V_Lyapunov buoy velocity/Smooth channel switching1/C2 transition/record C1_0 ==
  In1 : Inport
  Trigger : TriggerPort  VariantControl=Variant
  Out1 : Outport
  wires:
  In1/1 -> Out1/1

== system Marine_LocoMotive_UAV_est_git/UAV controller/u_r_V_Lyapunov buoy velocity/Smooth channel switching1/C2 transition/smooth transition to C1 ==
  In1 : Inport
  reset : Inport  Port=2
  Enable : EnablePort
  Discrete Transfer Fcn1 : DiscreteTransferFcn  Numerator=Bm_coup_LPF  Denominator=Am_coup_LPF  ExternalReset=Either
      settings: InputPortMap=u0,r7
  Out1 : Outport
  wires:
  reset/1 -> Discrete Transfer Fcn1/2
  In1/1 -> Discrete Transfer Fcn1/1
  Discrete Transfer Fcn1/1 -> Out1/1

== system Marine_LocoMotive_UAV_est_git/UAV controller/u_r_V_Lyapunov buoy velocity/Smooth channel switching1/C2 transition/trigger and reset latch ==
  trigger : Inport
  In2 : Inport  Port=2
  Abs : Abs
  Add : Sum
  Data Type Conversion : DataTypeConversion
  Data Type Conversion1 : DataTypeConversion
  Discrete Derivative1 : simulink/Discrete/Discrete Derivative  gainval=1.0  ICPrevScaledInput=0.0  OutMin=[]  OutMax=[]  OutDataType=fixdt(1, 16)  OutScaling=2^-10  DoSatur=off
  IC1 : InitialCondition  Value=0
  Saturation : Saturate  UpperLimit=1  LowerLimit=0
  Out1 : Outport
  wires:
  IC1/1 -> Saturation/1
  Data Type Conversion1/1 -> Discrete Derivative1/1
  Discrete Derivative1/1 -> Abs/1
  Saturation/1 -> Add/1
  In2/1 -> Data Type Conversion/1
  Data Type Conversion/1 -> Add/2
  Abs/1 -> IC1/1
  Add/1 -> Out1/1
  trigger/1 -> Data Type Conversion1/1

== matlab function Marine_LocoMotive_UAV_est_git/UAV controller/Coupling /u_a switch/MATLAB Function ==
  data: u_a input; u_a_out output; alpha input; theta_u input; m_q input; g input; c output
function [u_a_out,c] = fcn(u_a, alpha, theta_u, m_q, g)

threshold = m_q*g*cos(alpha);
c = 0;
if alpha <= pi/2
    if u_a <= threshold
        if (alpha + theta_u) < pi/2
            u_a_out = max(u_a, threshold);
            c = 1;
        else
            u_a_out = u_a;
        end
    else 
        if (alpha + theta_u) > pi/2
            u_a_out = 0;
            c = 1;
        else 
            u_a_out = u_a;
        end
    end
    
else % alpha > pi/2
    if u_a >= threshold
        if (alpha + theta_u) > pi/2
            u_a_out = max(u_a, threshold);
            c = 1;
        else
            u_a_out = u_a;
        end
    else 
        if (alpha + theta_u) < pi/2
            u_a_out = 0;
            c = 1;
        else 
            u_a_out = u_a;
        end
    end    
end

== matlab function Marine_LocoMotive_UAV_est_git/Quadrotor+buoy/3-DOF equations of motion Earth frame/Coupling state/MATLAB Function ==
  data: pos_T input; is_coupled output; re_couple input; coupled input; c output
function [is_coupled,c] = fcn(pos_T, re_couple, coupled)

% persistent coupled
% if isempty(coupled) 
%     coupled = 1;
% end

if and(pos_T == 1 , coupled == 1)
    coupled = 1;
    c = 1; 
    
elseif and(pos_T == 0 , coupled == 1)
    coupled = 0;
    c = 2;
elseif and(coupled == 0 , re_couple == 0)
    coupled = 0;
    c = 3;
elseif and(coupled == 0 , re_couple == 1)
    coupled = 1;
    c = 4;
elseif and(pos_T == 0 , coupled == 0)
    coupled = 0;
    c = 5;
else
    coupled = 1;
    c = 6;
end
    
is_coupled = coupled;

== matlab function Marine_LocoMotive_UAV_est_git/UAV controller/Coupling /Subsystem2/MATLAB Function ==
  data: u_a input; u_a_out output; alpha input; theta_u input; m_q input; g input
function u_a_out = fcn(u_a, alpha, theta_u, m_q, g)

threshold = m_q*g*cos(alpha);

if alpha <= pi/2
    if u_a <= threshold
        if (alpha + theta_u) < pi/2
            u_a_out = max(u_a, threshold)
        else
            u_a_out = u_a;
        end
    else 
        if (alpha + theta_u) > pi/2
            u_a_out = 0;
        else 
            u_a_out = u_a;
        end
    end
    
else % alpha > pi/2
    if u_a >= threshold
        if (alpha + theta_u) > pi/2
            u_a_out = max(u_a, threshold)
        else
            u_a_out = u_a;
        end
    else 
        if (alpha + theta_u) < pi/2
            u_a_out = 0;
        else 
            u_a_out = u_a;
        end
    end    
end

== matlab function Marine_LocoMotive_UAV_est_git/Sensors and Filters/Data processing/Estimate Attitude/Kalman Filter - Pitch ==
  settings: updateMethod=DISCRETE  sampleTime=T
  data: angle output; acc_angle input; gyro_rate input; opti_angle input; dt input
function angle   = fcn(acc_angle,gyro_rate,opti_angle,dt)
%#eml
    % a bias in the accelerometer will result in a bias in the filter
    % estimate
    Q_angle = 0.001;
    Q_gyro   = 0.001; %0.01;  %0.003
    R_angle  =  0.01;  %0.03

    
    persistent P_00;
    persistent P_01;
    persistent P_10;
    persistent P_11;
    persistent x_angle;
    persistent x_bias;
        
    if isempty(P_00)
        P_00 = 1.5*10^-4;
    end
    
    if isempty(P_01)
        P_01 = -1.4*10^-4;
    end
    if isempty(P_10)
        P_10 = -1.4*10^-4;
    end
    if isempty(P_11)
        P_11 = 11.4*10^-4;
    end
     if isempty(x_bias)
        x_bias = 0;
     end
     if isempty(x_angle)
        x_angle = 0;
     end
    
    
    % Calculate the new output
    x_angle = x_angle + dt * (gyro_rate - x_bias);%
    P_00 = P_00 -  dt * (P_10 + P_01) + Q_angle * dt;
    P_01 = P_01  - dt * P_11;
    P_10 = P_10  - dt * P_11;
    P_11 = P_11  + Q_gyro * dt;

    % Assuming H = [0.98 (effect of gyro) 0.02 (effect of acc)]
    %e = (0.97*x_angle + 0.03*acc_angle) - x_angle;
    e = (0.9*x_angle + 0.001*acc_angle + 0.099*opti_angle) - x_angle;
    S = P_00 + R_angle;
    K_0 = P_00 / S;
    K_1 = P_10 / S;

    % Correction
    x_angle = x_angle+  K_0 * e;
    x_bias  = x_bias+  K_1 * e;
    P_00 = P_00 - K_0 * P_00;
    P_01 = P_01 - K_0 * P_01;
    P_10 = P_10 - K_1 * P_00;
    P_11 = P_11 - K_1 * P_01;

    angle = x_angle;
%     P = [P_00 P_01; P_10 P_11];

== matlab function Marine_LocoMotive_UAV_est_git/Sensors and Filters/Coupling detection by r/Coupling state/MATLAB Function ==
  data: pos_T input; is_coupled output; re_couple input; coupled input; c output
function [is_coupled,c] = fcn(pos_T, re_couple, coupled)

% persistent coupled
% if isempty(coupled) 
%     coupled = 1;
% end

if and(pos_T == 1 , coupled == 1)
    coupled = 1;
    c = 1; 
    
elseif and(pos_T == 0 , coupled == 1)
    coupled = 0;
    c = 2;
elseif and(coupled == 0 , re_couple == 0)
    coupled = 0;
    c = 3;
elseif and(coupled == 0 , re_couple == 1)
    coupled = 1;
    c = 4;
elseif and(pos_T == 0 , coupled == 0)
    coupled = 0;
    c = 5;
else
    coupled = 1;
    c = 6;
end
    
is_coupled = coupled;

== matlab function Marine_LocoMotive_UAV_est_git/Sensors and Filters/Data processing/Estimate Position/Extrapolation - x ==
  settings: updateMethod=DISCRETE
  data: xin input; xout output; xdotin input; dt input; new input; isTracking input; x0 input
function xout = fcn(xin, xdotin, dt, new, isTracking,x0)
%#codegen

%
% Pass through input if "new" data available and OptiTrack is tracking.
% Otherwise, use linear interpolation to estimate the signal value and
% ignore the input data.
%
persistent x;

if( isempty(x) )
    x = x0;
end;

if( new == 1 && isTracking == 1 )
    x = xin;
else
    x = x+dt*xdotin;
end;

xout = x;

== matlab function Marine_LocoMotive_UAV_est_git/Refenrence Commands/setpoint velocity controller ==
  settings: updateMethod=DISCRETE
  data: eps input; r input; er_thr input; V_bar_out output; Lc0 input; c output; V0_bar input; V input
function [V_bar_out,c] = fcn(eps,r, er_thr, Lc0, V0_bar, V)%,...
            %c_sm, reset)

persistent V0_old
if isempty(V0_old) 
    V0_old = 0;
end

eps = abs(eps); % make sure that eps is positive.

% Velocity error is low, no output.
if (V0_bar - V <  eps) && (V0_bar - V >=  0)
    V_bar_out = V0_old;
    % return previous V0
    c = 0; 
% Velocity error is high, output the velocity only if the UAV is ready.
elseif (V0_bar - V >=  eps) && (Lc0 - r < er_thr)
    V_bar_out = V0_bar;
    % follow new V0
    c = 1;     
% Velocity error is low, no output.
elseif (V0_bar - V >  -eps) && (V0_bar - V <  0)
    V_bar_out = V0_old;
    % return previous V0
    c = 2; 
% Velocity error is high, output the velocity only if the UAV is ready.
elseif (V0_bar - V <=  -eps) && (Lc0 - r < er_thr)
    V_bar_out = V0_bar;
    % follow new V0
    c = 3;
else  % Velocity error is high, but UAV is not ready
    V_bar_out = V0_old;
    c = 4;
end

% when the new reference velocity is sent to the ouptut,
% set the old reference velocity to the current reference velocty
% to be the zero point when the reference velocty changes again.
if  V_bar_out == V0_bar
    V0_old = V0_bar;
end

== matlab function Marine_LocoMotive_UAV_est_git/Sensors and Filters/Data processing/Estimate Position/Extrapolation - z ==
  settings: updateMethod=DISCRETE  sampleTime=T
  data: xin input; xout output; xdotin input; dt input; new input; isTracking input; x0 input
function xout = fcn(xin, xdotin, dt, new, isTracking,x0)
%#codegen

%
% Pass through input if "new" data available and OptiTrack is tracking.
% Otherwise, use linear interpolation to estimate the signal value and
% ignore the input data.
%
persistent x;

if( isempty(x) )
    x = x0;
end

if( new == 1 && isTracking == 1 )
    x = xin;
else
    x = x+dt*xdotin;
end

xout = x;

== matlab function Marine_LocoMotive_UAV_est_git/UAV controller/cond1/MATLAB Function ==
  settings: updateMethod=DISCRETE
  data: r input; r_dot input; y output; coupled input; Lc input; dt input; t output
function [y,t]  = fcn(r,r_dot,coupled,Lc,dt)

persistent key
persistent timer

if isempty(key)
    key = 0;
end

if isempty(timer)
    timer = 0;
end

if (r > Lc - 0.1) && (r_dot > 0.25) && (key == 0)
    key = 1;
end

if (r < Lc - 0.12) && (r_dot < -0.1) && (key == 1)
    key = 0;
end

if (key == 1) && (coupled == 1)
    timer = timer + dt;
end

if (timer >= 1) % reset
    key = 0;
    timer = 0;
end

y = key;
t = timer;

== matlab function Marine_LocoMotive_UAV_est_git/UAV controller/u_a_Lyapunov/Subsystem1/cond1/MATLAB Function ==
  data: r input; r_dot input; y output; coupled input; Lc input; dt input; t output
function [y,t]  = fcn(r,r_dot,coupled,Lc,dt)

persistent key
persistent timer

if isempty(key)
    key = 0;
end

if isempty(timer)
    timer = 0;
end

if (r > Lc - 0.1) && (r_dot > 0.25) && (key == 0)
    key = 1;
end

if (r < Lc - 0.12) && (r_dot < -0.1) && (key == 1)
    key = 0;
end

if (key == 1) && (coupled == 1)
    timer = timer + dt;
end

if (timer >= 1) % reset
    key = 0;
    timer = 0;
end

y = key;
t = timer;
